simulink model "VMC_3D_Quad_trot"  (R2017a)
settings: Solver=VariableStepAuto  StartTime=0.0  StopTime=20  RelTol=1e-3
model workspace (MATLAB code in the model file):
  | npt=4;  % 接触点个数
  | model = batery_quadruped(npt);
  | f0=zeros(6,1);
  | vx_init=0;
  | x_init = [1;0;0;0; 0;0;1.1; 0;0;0;...
  |           vx_init;0;0]; % initial state
  | q_init = [0;0.5857;-1.1714;0;0.5857;-1.1714;...
  |           0;0.5857;-1.1714;0;0.5857;-1.1714];
  | %q_init = [0;0.7227;-1.4454;0;0.7227;-1.4454;...
  |  %         0;0.7227;-1.4454;0;0.7227;-1.4454];
  | %qd_init= [-2.061;-0.4906];
undefined symbols (not defined in the file or in its folder): batery_quadruped, CalHipVel, CalState, fbanim, FootPUnderHip, Fpt, GaitGenerator, gcontact, gcPosVel, LateralForce, VMC3D
libraries: simulink x4
settings Model: Creator=Jack Lee  LastModifiedBy=jackLee

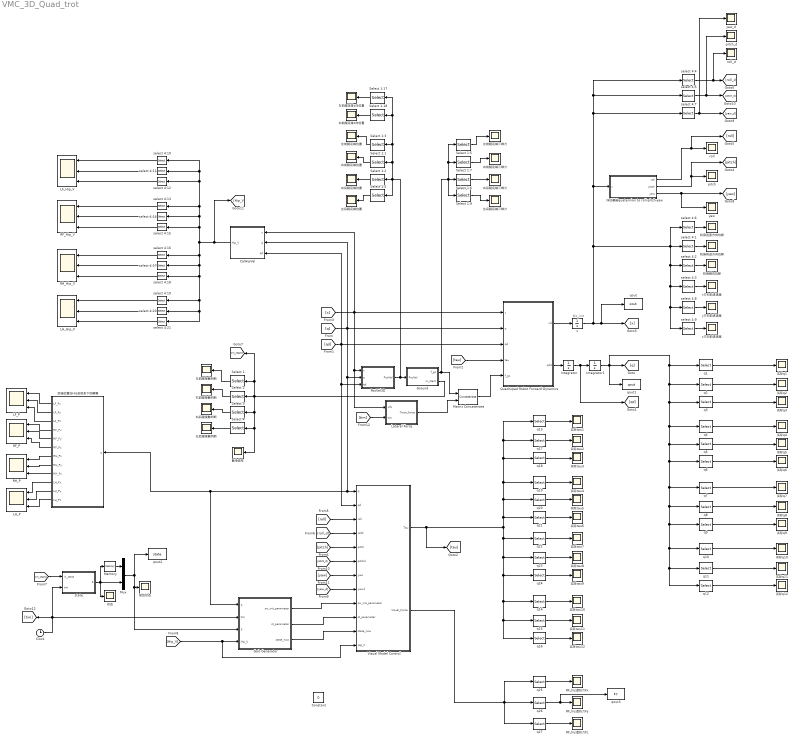
== system VMC_3D_Quad_trot ==
  note: 有x_init
  CalHipVel : Subsystem
  Clock : Clock
  Constant : Constant  Value=0
  Gait Generator : Subsystem
  Ground : Subsystem
  Integrator : Integrator
  Integrator1 : Integrator  InitialCondition=q_init
  LF_Hip_V : Scope  NumInputPorts=3
  LF_P : Scope  NumInputPorts=3
  LH_Hip_V : Scope  NumInputPorts=3
  LH_P : Scope  NumInputPorts=3
  Lateral Force : Subsystem
  Matrix Concatenate : Concatenate  Mode=Multidimensional array  ConcatenateDimension=2
  Memory : Memory  X0=4
  Mux : Mux  Inputs=2
  PosVel3D : Subsystem
  Quadruped Robot Forward Dynamics : Subsystem
  RF_Hip_V : Scope  NumInputPorts=3
  RF_P : Scope  NumInputPorts=3
  RF_hip虚拟力Fx : Scope
  RF_hip虚拟力Fy : Scope
  RF_hip虚拟力Fz : Scope
  RH_Hip_V : Scope  NumInputPorts=3
  RH_P : Scope  NumInputPorts=3
  Select 1 : Selector  InputPortWidth=4  IndexOptions=Index vector (dialog)  Indices=[1]  OutputSizes=1
  Select 1:1 : Selector  NumberOfDimensions=2  InputPortWidth=6  IndexOptions=Index vector (dialog),Index vector (dialog)  Indices=[1 2 3],2  OutputSizes=1,1
  Select 1:17 : Selector  NumberOfDimensions=2  InputPortWidth=6  IndexOptions=Index vector (dialog),Index vector (dialog)  Indices=[3],1  OutputSizes=1,1
  Select 1:18 : Selector  NumberOfDimensions=2  InputPortWidth=6  IndexOptions=Index vector (dialog),Index vector (dialog)  Indices=[3],2  OutputSizes=1,1
  Select 1:2 : Selector  NumberOfDimensions=2  InputPortWidth=6  IndexOptions=Index vector (dialog),Index vector (dialog)  Indices=[1 2 3],3  OutputSizes=1,1
  Select 1:3 : Selector  NumberOfDimensions=2  InputPortWidth=6  IndexOptions=Index vector (dialog),Index vector (dialog)  Indices=[1 2 3],1  OutputSizes=1,1
  Select 1:4 : Selector  NumberOfDimensions=2  InputPortWidth=6  IndexOptions=Index vector (dialog),Index vector (dialog)  Indices=[1 2 3],4  OutputSizes=1,1
  Select 1:5 : Selector  NumberOfDimensions=2  InputPortWidth=6  IndexOptions=Index vector (dialog),Index vector (dialog)  Indices=[4 5 6],1  OutputSizes=1,1
  Select 1:6 : Selector  NumberOfDimensions=2  InputPortWidth=6  IndexOptions=Index vector (dialog),Index vector (dialog)  Indices=[4 5 6],3  OutputSizes=1,1
  Select 1:7 : Selector  NumberOfDimensions=2  InputPortWidth=6  IndexOptions=Index vector (dialog),Index vector (dialog)  Indices=[4 5 6],2  OutputSizes=1,1
  Select 1:9 : Selector  NumberOfDimensions=2  InputPortWidth=6  IndexOptions=Index vector (dialog),Index vector (dialog)  Indices=[4 5 6],4  OutputSizes=1,1
  Select 2 : Selector  InputPortWidth=4  IndexOptions=Index vector (dialog)  Indices=[2]  OutputSizes=1
  Select 3 : Selector  InputPortWidth=4  IndexOptions=Index vector (dialog)  Indices=[3]  OutputSizes=1
  Select 4 : Selector  InputPortWidth=4  IndexOptions=Index vector (dialog)  Indices=[4]  OutputSizes=1
  Visual Model Control : Subsystem
  pitch : Scope
  pitch_d : Scope
  q1 : Selector  InputPortWidth=12  IndexOptions=Index vector (dialog)  Indices=1  OutputSizes=1
  q10 : Selector  InputPortWidth=12  IndexOptions=Index vector (dialog)  Indices=10  OutputSizes=1
  q11 : Selector  InputPortWidth=12  IndexOptions=Index vector (dialog)  Indices=11  OutputSizes=1
  q12 : Selector  InputPortWidth=12  IndexOptions=Index vector (dialog)  Indices=12  OutputSizes=1
  q13 : Selector  InputPortWidth=12  IndexOptions=Index vector (dialog)  Indices=1  OutputSizes=1
  q14 : Selector  InputPortWidth=12  IndexOptions=Index vector (dialog)  Indices=10  OutputSizes=1
  q15 : Selector  InputPortWidth=12  IndexOptions=Index vector (dialog)  Indices=11  OutputSizes=1
  q16 : Selector  InputPortWidth=12  IndexOptions=Index vector (dialog)  Indices=12  OutputSizes=1
  q17 : Selector  InputPortWidth=12  IndexOptions=Index vector (dialog)  Indices=2  OutputSizes=1
  q18 : Selector  InputPortWidth=12  IndexOptions=Index vector (dialog)  Indices=3  OutputSizes=1
  q19 : Selector  InputPortWidth=12  IndexOptions=Index vector (dialog)  Indices=4  OutputSizes=1
  q2 : Selector  InputPortWidth=12  IndexOptions=Index vector (dialog)  Indices=2  OutputSizes=1
  q20 : Selector  InputPortWidth=12  IndexOptions=Index vector (dialog)  Indices=5  OutputSizes=1
  q21 : Selector  InputPortWidth=12  IndexOptions=Index vector (dialog)  Indices=6  OutputSizes=1
  q22 : Selector  InputPortWidth=12  IndexOptions=Index vector (dialog)  Indices=7  OutputSizes=1
  q23 : Selector  InputPortWidth=12  IndexOptions=Index vector (dialog)  Indices=8  OutputSizes=1
  q24 : Selector  InputPortWidth=12  IndexOptions=Index vector (dialog)  Indices=9  OutputSizes=1
  q25 : Selector  InputPortWidth=12  IndexOptions=Index vector (dialog)  Indices=4  OutputSizes=1
  q26 : Selector  InputPortWidth=12  IndexOptions=Index vector (dialog)  Indices=5  OutputSizes=1
  q27 : Selector  InputPortWidth=12  IndexOptions=Index vector (dialog)  Indices=6  OutputSizes=1
  q3 : Selector  InputPortWidth=12  IndexOptions=Index vector (dialog)  Indices=3  OutputSizes=1
  q4 : Selector  InputPortWidth=12  IndexOptions=Index vector (dialog)  Indices=4  OutputSizes=1
  q5 : Selector  InputPortWidth=12  IndexOptions=Index vector (dialog)  Indices=5  OutputSizes=1
  q6 : Selector  InputPortWidth=12  IndexOptions=Index vector (dialog)  Indices=6  OutputSizes=1
  q7 : Selector  InputPortWidth=12  IndexOptions=Index vector (dialog)  Indices=7  OutputSizes=1
  q8 : Selector  InputPortWidth=12  IndexOptions=Index vector (dialog)  Indices=8  OutputSizes=1
  q9 : Selector  InputPortWidth=12  IndexOptions=Index vector (dialog)  Indices=9  OutputSizes=1
  qout : ToWorkspace  VariableName=xout  SampleTime=-1
  qout1 : ToWorkspace  VariableName=qout  SampleTime=-1
  qout2 : ToWorkspace  VariableName=state  SampleTime=-1
  qout3 : ToWorkspace  VariableName=FY  SampleTime=-1
  roll : Scope
  roll_d : Scope
  select 4:1 : Selector  InputPortWidth=13  IndexOptions=Index vector (dialog)  Indices=[5]  OutputSizes=1
  select 4:10 : Selector  InputPortWidth=12  IndexOptions=Index vector (dialog)  Indices=[1]  OutputSizes=1
  select 4:11 : Selector  InputPortWidth=12  IndexOptions=Index vector (dialog)  Indices=[2]  OutputSizes=1
  select 4:12 : Selector  InputPortWidth=12  IndexOptions=Index vector (dialog)  Indices=[3]  OutputSizes=1
  select 4:13 : Selector  InputPortWidth=12  IndexOptions=Index vector (dialog)  Indices=[4]  OutputSizes=1
  select 4:14 : Selector  InputPortWidth=12  IndexOptions=Index vector (dialog)  Indices=[5]  OutputSizes=1
  select 4:15 : Selector  InputPortWidth=12  IndexOptions=Index vector (dialog)  Indices=[6]  OutputSizes=1
  select 4:16 : Selector  InputPortWidth=12  IndexOptions=Index vector (dialog)  Indices=[7]  OutputSizes=1
  select 4:17 : Selector  InputPortWidth=12  IndexOptions=Index vector (dialog)  Indices=[8]  OutputSizes=1
  select 4:18 : Selector  InputPortWidth=12  IndexOptions=Index vector (dialog)  Indices=[9]  OutputSizes=1
  select 4:19 : Selector  InputPortWidth=12  IndexOptions=Index vector (dialog)  Indices=[10]  OutputSizes=1
  select 4:2 : Selector  InputPortWidth=13  IndexOptions=Index vector (dialog)  Indices=[6]  OutputSizes=1
  select 4:20 : Selector  InputPortWidth=12  IndexOptions=Index vector (dialog)  Indices=[11]  OutputSizes=1
  select 4:21 : Selector  InputPortWidth=12  IndexOptions=Index vector (dialog)  Indices=[12]  OutputSizes=1
  select 4:3 : Selector  InputPortWidth=13  IndexOptions=Index vector (dialog)  Indices=[11]  OutputSizes=1
  select 4:4 : Selector  InputPortWidth=13  IndexOptions=Index vector (dialog)  Indices=[8]  OutputSizes=1
  select 4:5 : Selector  InputPortWidth=13  IndexOptions=Index vector (dialog)  Indices=[9]  OutputSizes=1
  select 4:6 : Selector  InputPortWidth=13  IndexOptions=Index vector (dialog)  Indices=[7]  OutputSizes=1
  select 4:7 : Selector  InputPortWidth=13  IndexOptions=Index vector (dialog)  Indices=[10]  OutputSizes=1
  select 4:8 : Selector  InputPortWidth=13  IndexOptions=Index vector (dialog)  Indices=[12]  OutputSizes=1
  select 4:9 : Selector  InputPortWidth=13  IndexOptions=Index vector (dialog)  Indices=[13]  OutputSizes=1
  state : Subsystem
  x : Integrator  InitialCondition=x_init
  x方向前进速度 : Scope
  yaw : Scope
  yaw_d : Scope
  y方向前进速度 : Scope
  z方向前进速度 : Scope
  前后状态 : Scope
  右前腿接触判断 : Scope
  右前腿足端z向位置 : Scope
  右前腿足端三维力 : Scope
  右前腿足端位置 : Scope
  右后腿接触判断 : Scope
  右后腿足端三维力 : Scope
  右后腿足端位置 : Scope
  实际q{1..12} (12 alike) : Scope
  实际tau{1..12} (12 alike) : Scope
  左前腿接触判断 : Scope
  左前腿足端z向位置 : Scope
  左前腿足端三维力 : Scope
  左前腿足端位置 : Scope
  左后腿接触判断 : Scope
  左后腿足端三维力 : Scope
  左后腿足端位置 : Scope
  机身侧向位移 : Scope
  机身前进方向位移 : Scope
  机身竖直方向位移 : Scope
  浮动基座quaternion to roll-pitch-yaw : Subsystem
  状态 : Scope
  触地信号 : Scope
  足端位置在Hip坐标系下的解算 : Subsystem
  wires:
  Quadruped Robot Forward Dynamics/1(xd) -> x/1
  Quadruped Robot Forward Dynamics/2(qdd) -> Integrator/1
  Integrator/1 -> [qd], Integrator1/1
  Ground/1(f_gc) -> Select 1:5/1, Select 1:7/1, Select 1:9/1, Select 1:6/1, Matrix Concatenate/1
  [tau] -> Quadruped Robot Forward Dynamics/4(tau)
  x/1 -> select 4:5/1, select 4:4/1, select 4:7/1, 浮动基座quaternion to roll-pitch-yaw/1(x), select 4:9/1, select 4:8/1, select 4:3/1, select 4:2/1, select 4:6/1, select 4:1/1, qout/1, [x]
  Ground/2(in_ctact) -> [in_ctact], Select 1/1, 触地信号/1, Select 4/1, Select 3/1, Select 2/1
  [x] -> CalHipVel/1(x), Lateral Force/1(xfb), PosVel3D/1(x), Quadruped Robot Forward Dynamics/1(x)
  [qd] -> CalHipVel/3(qd), Visual Model Control/2(qd), PosVel3D/3(qd), Quadruped Robot Forward Dynamics/3(qd)
  PosVel3D/1(PosVel) -> Select 1:18/1, Select 1:17/1, Select 1:3/1, Select 1:1/1, Select 1:4/1, Select 1:2/1, Ground/1(PosVel)
  Select 1:2/1 -> 右后腿足端位置/1
  Select 1:4/1 -> 左后腿足端位置/1
  Select 1:1/1 -> 右前腿足端位置/1
  Select 1:3/1 -> 左前腿足端位置/1
  Select 1:5/1 -> 左前腿足端三维力/1
  Select 1:7/1 -> 右前腿足端三维力/1
  Select 1:6/1 -> 右后腿足端三维力/1
  Select 1:9/1 -> 左后腿足端三维力/1
  Select 1/1 -> 左前腿接触判断/1
  Select 2/1 -> 右前腿接触判断/1
  Select 3/1 -> 右后腿接触判断/1
  Select 4/1 -> 左后腿接触判断/1
  select 4:6/1 -> 机身竖直方向位移/1
  q12/1 -> 实际q12/1
  q11/1 -> 实际q11/1
  q10/1 -> 实际q10/1
  q9/1 -> 实际q9/1
  q8/1 -> 实际q8/1
  q7/1 -> 实际q7/1
  q6/1 -> 实际q6/1
  q5/1 -> 实际q5/1
  q4/1 -> 实际q4/1
  q3/1 -> 实际q3/1
  q2/1 -> 实际q2/1
  Integrator1/1 -> q12/1, q11/1, q10/1, q9/1, q8/1, q7/1, q6/1, q5/1, q4/1, q3/1, q2/1, q1/1, qout1/1, [q]
  q18/1 -> 实际tau3/1
  q24/1 -> 实际tau9/1
  q22/1 -> 实际tau7/1
  q16/1 -> 实际tau12/1
  q17/1 -> 实际tau2/1
  q20/1 -> 实际tau5/1
  q21/1 -> 实际tau6/1
  q23/1 -> 实际tau8/1
  Visual Model Control/1(Tau) -> [tau], q16/1, q15/1, q14/1, q24/1, q23/1, q22/1, q13/1, q17/1, q18/1, q19/1, q20/1, q21/1
  q14/1 -> 实际tau10/1
  q19/1 -> 实际tau4/1
  q13/1 -> 实际tau1/1
  q15/1 -> 实际tau11/1
  select 4:1/1 -> 机身前进方向位移/1
  Select 1:18/1 -> 右前腿足端z向位置/1
  Select 1:17/1 -> 左前腿足端z向位置/1
  select 4:3/1 -> x方向前进速度/1
  浮动基座quaternion to roll-pitch-yaw/2(pitch) -> [pitch], pitch/1
  浮动基座quaternion to roll-pitch-yaw/1(roll) -> [roll], roll/1
  浮动基座quaternion to roll-pitch-yaw/3(yaw) -> [yaw], yaw/1
  select 4:4/1 -> roll_d/1, [roll_d]
  q1/1 -> 实际q1/1
  [in_ctact] -> state/1(in_ctact)
  state/1(S) -> Memory/1, Mux/2, 状态/1
  select 4:5/1 -> pitch_d/1, [pitch_d]
  select 4:7/1 -> yaw_d/1, [yaw_d]
  [roll] -> Visual Model Control/3(roll)
  [roll_d] -> Visual Model Control/4(rolld)
  [pitch] -> Visual Model Control/5(pitch)
  [Hip_V] -> Visual Model Control/12(Hip_V), Gait Generator/4(Hip_V)
  [q] -> CalHipVel/2(q), Gait Generator/1(q), 足端位置在Hip坐标系下的解算/1(q), Visual Model Control/1(q), PosVel3D/2(q), Quadruped Robot Forward Dynamics/2(q)
  Gait Generator/1(sw_init_parameter) -> Visual Model Control/9(sw_init_parameter)
  Gait Generator/2(st_parameter) -> Visual Model Control/10(st_parameter)
  Gait Generator/3(state_now) -> Visual Model Control/11(state_now)
  Clock/1 -> [tim], state/2(tim), Gait Generator/2(tim)
  Mux/1 -> qout2/1, 前后状态/1, Gait Generator/3(S)
  Memory/1 -> Mux/1
  [yaw_d] -> Visual Model Control/8(yawd)
  [pitch_d] -> Visual Model Control/6(pitchd)
  [yaw] -> Visual Model Control/7(yaw)
  select 4:9/1 -> z方向前进速度/1
  足端位置在Hip坐标系下的解算/1(LF_Px) -> LF_P/1
  足端位置在Hip坐标系下的解算/2(LF_Py) -> LF_P/2
  足端位置在Hip坐标系下的解算/3(LF_Pz) -> LF_P/3
  足端位置在Hip坐标系下的解算/4(RF_Px) -> RF_P/1
  足端位置在Hip坐标系下的解算/5(RF_Py) -> RF_P/2
  足端位置在Hip坐标系下的解算/6(RF_Pz) -> RF_P/3
  足端位置在Hip坐标系下的解算/7(RH_Px) -> RH_P/1
  足端位置在Hip坐标系下的解算/8(RH_Py) -> RH_P/2
  足端位置在Hip坐标系下的解算/9(RH_Pz) -> RH_P/3
  足端位置在Hip坐标系下的解算/12(LH_Pz) -> LH_P/3
  足端位置在Hip坐标系下的解算/11(LH_Py) -> LH_P/2
  足端位置在Hip坐标系下的解算/10(LH_Px) -> LH_P/1
  select 4:2/1 -> 机身侧向位移/1
  select 4:8/1 -> y方向前进速度/1
  select 4:10/1 -> LF_Hip_V/1
  select 4:12/1 -> LF_Hip_V/3
  select 4:11/1 -> LF_Hip_V/2
  select 4:15/1 -> RF_Hip_V/3
  select 4:13/1 -> RF_Hip_V/1
  select 4:14/1 -> RF_Hip_V/2
  select 4:18/1 -> RH_Hip_V/3
  select 4:16/1 -> RH_Hip_V/1
  select 4:17/1 -> RH_Hip_V/2
  select 4:21/1 -> LH_Hip_V/3
  select 4:19/1 -> LH_Hip_V/1
  CalHipVel/1(Hip_V) -> [Hip_V], select 4:15/1, select 4:13/1, select 4:12/1, select 4:11/1, select 4:10/1, select 4:14/1, select 4:17/1, select 4:18/1, select 4:19/1, select 4:20/1, select 4:21/1, select 4:16/1
  select 4:20/1 -> LH_Hip_V/2
  [tim] -> Lateral Force/2(tim)
  Lateral Force/1(Torso_force) -> Matrix Concatenate/2
  Matrix Concatenate/1 -> Quadruped Robot Forward Dynamics/5(f_gc)
  Visual Model Control/2(Visual_Force) -> q27/1, q25/1, q26/1
  q27/1 -> RF_hip虚拟力Fz/1
  q26/1 -> qout3/1, RF_hip虚拟力Fy/1
  q25/1 -> RF_hip虚拟力Fx/1

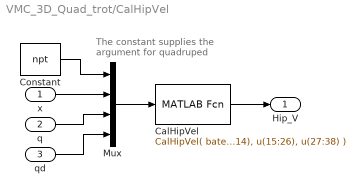
== system VMC_3D_Quad_trot/CalHipVel ==
  note: The constant supplies the
      | argument for quadruped
  x : Inport
  q : Inport  Port=2
  qd : Inport  Port=3
  CalHipVel : MATLABFcn  MATLABFcn=CalHipVel( batery_quadruped(u(1)), u(2:14), u(15:26), u(27:38) )  OutputDimensions=[12 1]  OutputSignalType=real  Output1D=off
  Constant : Constant  Value=npt
  Mux : Mux
  Hip_V : Outport
  wires:
  CalHipVel/1 -> Hip_V/1
  Mux/1 -> CalHipVel/1
  x/1 -> Mux/2
  Constant/1 -> Mux/1
  q/1 -> Mux/3
  qd/1 -> Mux/4

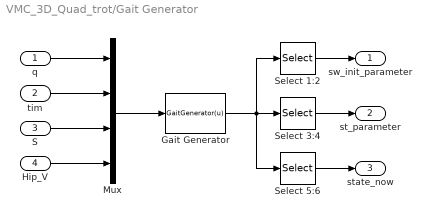
== system VMC_3D_Quad_trot/Gait Generator ==
  q : Inport
  tim : Inport  Port=2
  S : Inport  Port=3
  Hip_V : Inport  Port=4
  Gait Generator : MATLABFcn  MATLABFcn=GaitGenerator(u)  OutputDimensions=[32 1]  OutputSignalType=real  Output1D=off
  Mux : Mux
  Select 1:2 : Selector  InputPortWidth=32  IndexOptions=Index vector (dialog)  Indices=[1:21]  OutputSizes=1
  Select 3:4 : Selector  InputPortWidth=32  IndexOptions=Index vector (dialog)  Indices=[22:31]  OutputSizes=1
  Select 5:6 : Selector  InputPortWidth=32  IndexOptions=Index vector (dialog)  Indices=[32]  OutputSizes=1
  sw_init_parameter : Outport
  st_parameter : Outport  Port=2
  state_now : Outport  Port=3
  wires:
  q/1 -> Mux/1
  Select 1:2/1 -> sw_init_parameter/1
  Select 3:4/1 -> st_parameter/1
  Select 5:6/1 -> state_now/1
  Mux/1 -> Gait Generator/1
  Gait Generator/1 -> Select 5:6/1, Select 1:2/1, Select 3:4/1
  tim/1 -> Mux/2
  S/1 -> Mux/3
  Hip_V/1 -> Mux/4

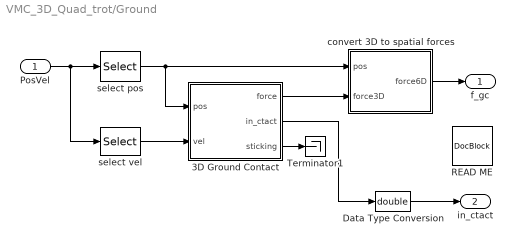
== system VMC_3D_Quad_trot/Ground ==
  PosVel : Inport
  3D Ground Contact : Subsystem  mask(3D Nonlinear Ground Contact with Friction){K=5e5, D=2000, mu=0.7, np=npt}
      mask prompts: K "Stiffness (K)"; D "Damping (D)"; mu "Coefficient of Friction (mu)"; np "Number of Contact Points"
      mask help:
      | Given two 3xnp arrays containing contact-point positions and
      | velocities, calculate the 3xnp array of ground-reaction forces
      | acting on those points. Also calculate 1xnp boolean vectors
      | in_ctact (true if normal force >0) and sticking (true if inside
      | or on boundary of friction cone).  Zero-crossing detection is
      | enabled at both make/break contact and stick/slip transitions.
  Data Type Conversion : DataTypeConversion  OutDataTypeStr=double
  READ ME : simulink/Model-Wide Utilities/DocBlock  DocumentType=Text
      content=|
      | This subsystem implements the Simulink ground-contact model in 3D.  The
      | input is a 6x(npt) matrix such that column i contains the 3D position (top
      | 3 elements) and linear velocity (bottom 3 elements) of ground-contact
      | point number i (i.e., the i^th point defined in the "gc" field of the
      | system model data structure).  The output is a 6x(npt) matrix such that
      | column i is the spatial force acting on point number i.  All quantities
      | are expressed in base (body 0) coordinates.
      |
      | The first thing that happens is that the input matrix is split into
      | separate position and velocity matrices.  Both are then sent to the "3D
      | Ground Contact" subsystem, which calculates the force acting on each
      | point.  The "force" output is a 3x(npt) matrix of linear forces, which is
      | converted to a matrix of spatial forces by the final block in the
      | subsystem.  The other two outputs are 1x(npt) arrays of Boolean variables
      | such that in_ctact(i) is true if point i is in contact with the ground
      | (meaning that it is experiencing a nonzero force) and sticking(i) is true
      | if point i is sticking (due to friction) to the ground.
      |
      | The subsystem "3D Ground Contact" is a masked subsystem.  If you
      | double-click on this block then you will get a dialog window displaying
      | the following parameters: Stiffness (K), Damping (D), coefficient of
      | friction (mu), and Number of Contact Points.  The first three must be
      | strictly-positive scalars, and the fourth must equal the number of points
      | defined in the "gc" field of the system model data structure.  The current
      | settings of K, D and mu correspond to a soft, very slippery plastic
      | surface.  Increasing K will make it harder, and increasing the ratio K/D
      | will make it bouncier, but be aware that both increase the stiffness of
      | the differential equations that Simulink is solving, meaning that Simulink
      | will be forced to take smaller steps.  A typical value of mu for a safe
      | (non-slip) floor is 0.5.
      |
      | To see how this subsystem is implemented, you will have to look under the
      | mask.  You can do that by right-clicking on the block and selecting the
      | menu option "Look Under Mask".  There, you will find that this block is
      | based on the function gcontact, and you will also find a bit more
      | documentation.
  Terminator1 : Terminator
  convert 3D to spatial forces : Subsystem
  select pos : Selector  NumberOfDimensions=2  InputPortWidth=3  IndexOptions=Index vector (dialog),Select all  Indices=[1 2 3],1  OutputSizes=1,1
  select vel : Selector  NumberOfDimensions=2  InputPortWidth=3  IndexOptions=Index vector (dialog),Select all  Indices=[4 5 6],1  OutputSizes=1,1
  f_gc : Outport
  in_ctact : Outport  Port=2
  wires:
  PosVel/1 -> select pos/1, select vel/1
  select pos/1 -> convert 3D to spatial forces/1(pos), 3D Ground Contact/1(pos)
  convert 3D to spatial forces/1(force6D) -> f_gc/1
  select vel/1 -> 3D Ground Contact/2(vel)
  3D Ground Contact/1(force) -> convert 3D to spatial forces/2(force3D)
  3D Ground Contact/3(sticking) -> Terminator1/1
  3D Ground Contact/2(in_ctact) -> Data Type Conversion/1
  Data Type Conversion/1 -> in_ctact/1

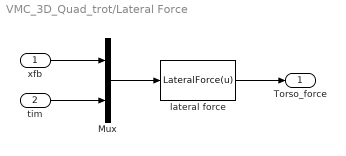
== system VMC_3D_Quad_trot/Lateral Force ==
  xfb : Inport
  tim : Inport  Port=2
  Mux : Mux  Inputs=2
  lateral force : MATLABFcn  MATLABFcn=LateralForce(u)  OutputDimensions=[6 1]  OutputSignalType=real  Output1D=off
  Torso_force : Outport
  wires:
  lateral force/1 -> Torso_force/1
  Mux/1 -> lateral force/1
  xfb/1 -> Mux/1
  tim/1 -> Mux/2

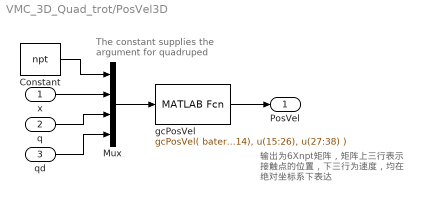
== system VMC_3D_Quad_trot/PosVel3D ==
  note: 输出为6Xnpt矩阵，矩阵上三行表示
      | 接触点的位置，下三行为速度，均在
      | 绝对坐标系下表达
  note: The constant supplies the
      | argument for quadruped
  x : Inport
  q : Inport  Port=2
  qd : Inport  Port=3
  Constant : Constant  Value=npt
  Mux : Mux
  gcPosVel : MATLABFcn  MATLABFcn=gcPosVel( batery_quadruped(u(1)), u(2:14), u(15:26), u(27:38) )  OutputDimensions=[6 npt]  OutputSignalType=real  Output1D=off
  PosVel : Outport
  wires:
  gcPosVel/1 -> PosVel/1
  Mux/1 -> gcPosVel/1
  x/1 -> Mux/2
  Constant/1 -> Mux/1
  q/1 -> Mux/3
  qd/1 -> Mux/4

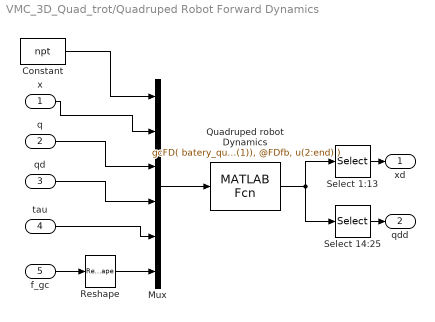
== system VMC_3D_Quad_trot/Quadruped Robot Forward Dynamics ==
  x : Inport
  q : Inport  Port=2
  qd : Inport  Port=3
  tau : Inport  Port=4
  f_gc : Inport  Port=5
  Constant : Constant  Value=npt
  Mux : Mux  Inputs=6
  Quadruped robot Dynamics : MATLABFcn  MATLABFcn=gcFD( batery_quadruped(u(1)), @FDfb, u(2:end) )  OutputDimensions=[25 1]  OutputSignalType=real  Output1D=off
  Reshape : Reshape  OutputDimensionality=Column vector (2-D)
  Select 14:25 : Selector  InputPortWidth=25  IndexOptions=Index vector (dialog)  Indices=[14 15 16 17 18 19 20 21 22 23 24 25]  OutputSizes=1
  Select 1:13 : Selector  InputPortWidth=25  IndexOptions=Index vector (dialog)  Indices=[1 2 3 4 5 6 7 8 9 10 11 12 13]  OutputSizes=1
  xd : Outport
  qdd : Outport  Port=2
  wires:
  f_gc/1 -> Reshape/1
  Mux/1 -> Quadruped robot Dynamics/1
  Reshape/1 -> Mux/6
  x/1 -> Mux/2
  Constant/1 -> Mux/1
  Select 14:25/1 -> qdd/1
  Select 1:13/1 -> xd/1
  Quadruped robot Dynamics/1 -> Select 14:25/1, Select 1:13/1
  q/1 -> Mux/3
  qd/1 -> Mux/4
  tau/1 -> Mux/5

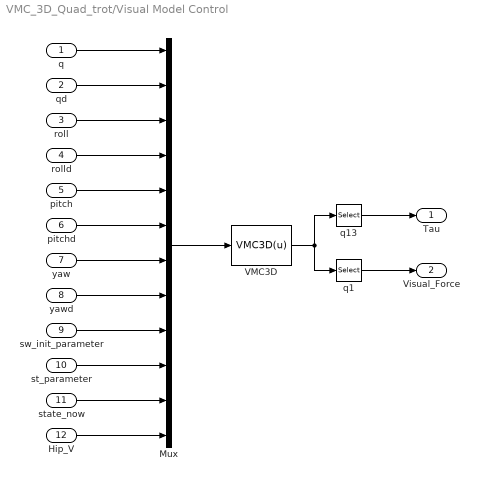
== system VMC_3D_Quad_trot/Visual Model Control ==
  q : Inport
  qd : Inport  Port=2
  roll : Inport  Port=3
  rolld : Inport  Port=4
  pitch : Inport  Port=5
  pitchd : Inport  Port=6
  yaw : Inport  Port=7
  yawd : Inport  Port=8
  sw_init_parameter : Inport  Port=9
  st_parameter : Inport  Port=10
  state_now : Inport  Port=11
  Hip_V : Inport  Port=12
  Mux : Mux  Inputs=12
  VMC3D : MATLABFcn  MATLABFcn=VMC3D(u)  OutputDimensions=[24 1]  OutputSignalType=real  Output1D=off
  q1 : Selector  InputPortWidth=24  IndexOptions=Index vector (dialog)  Indices=[13:24]  OutputSizes=1
  q13 : Selector  InputPortWidth=24  IndexOptions=Index vector (dialog)  Indices=[1:12]  OutputSizes=1
  Tau : Outport
  Visual_Force : Outport  Port=2
  wires:
  q/1 -> Mux/1
  roll/1 -> Mux/3
  pitch/1 -> Mux/5
  Mux/1 -> VMC3D/1
  qd/1 -> Mux/2
  rolld/1 -> Mux/4
  pitchd/1 -> Mux/6
  yaw/1 -> Mux/7
  yawd/1 -> Mux/8
  sw_init_parameter/1 -> Mux/9
  st_parameter/1 -> Mux/10
  state_now/1 -> Mux/11
  Hip_V/1 -> Mux/12
  q13/1 -> Tau/1
  q1/1 -> Visual_Force/1
  VMC3D/1 -> q13/1, q1/1

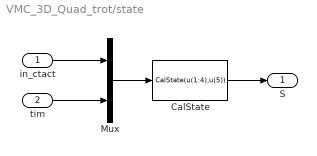
== system VMC_3D_Quad_trot/state ==
  in_ctact : Inport
  tim : Inport  Port=2
  CalState : MATLABFcn  MATLABFcn=CalState(u(1:4),u(5))  OutputDimensions=1  OutputSignalType=real  Output1D=off
  Mux : Mux  Inputs=2
  S : Outport
  wires:
  CalState/1 -> S/1
  Mux/1 -> CalState/1
  in_ctact/1 -> Mux/1
  tim/1 -> Mux/2

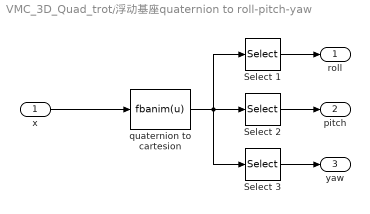
== system VMC_3D_Quad_trot/浮动基座quaternion to roll-pitch-yaw ==
  x : Inport
  Select 1 : Selector  InputPortWidth=6  IndexOptions=Index vector (dialog)  Indices=[4]  OutputSizes=1
  Select 2 : Selector  InputPortWidth=6  IndexOptions=Index vector (dialog)  Indices=[5]  OutputSizes=1
  Select 3 : Selector  InputPortWidth=6  IndexOptions=Index vector (dialog)  Indices=[6]  OutputSizes=1
  "quaternion to cartesion " : MATLABFcn  MATLABFcn=fbanim(u)  OutputDimensions=[6 1]  OutputSignalType=real  Output1D=off
  roll : Outport
  pitch : Outport  Port=2
  yaw : Outport  Port=3
  wires:
  x/1 -> "quaternion to cartesion "/1
  Select 1/1 -> roll/1
  Select 2/1 -> pitch/1
  "quaternion to cartesion "/1 -> Select 1/1, Select 3/1, Select 2/1
  Select 3/1 -> yaw/1

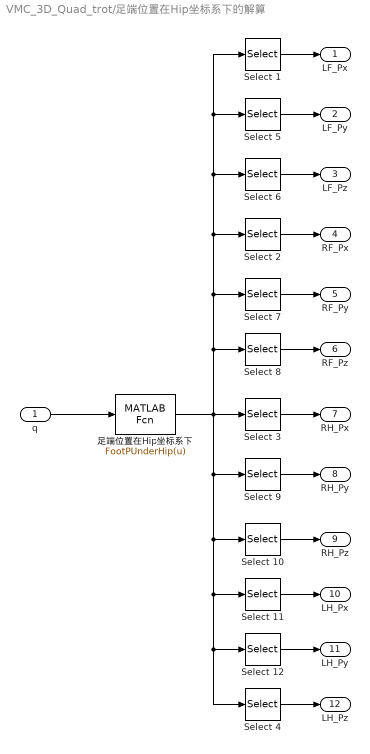
== system VMC_3D_Quad_trot/足端位置在Hip坐标系下的解算 ==
  q : Inport
  Select 1 : Selector  InputPortWidth=12  IndexOptions=Index vector (dialog)  Indices=[1]  OutputSizes=1
  Select 10 : Selector  InputPortWidth=12  IndexOptions=Index vector (dialog)  Indices=[9]  OutputSizes=1
  Select 11 : Selector  InputPortWidth=12  IndexOptions=Index vector (dialog)  Indices=[10]  OutputSizes=1
  Select 12 : Selector  InputPortWidth=12  IndexOptions=Index vector (dialog)  Indices=[11]  OutputSizes=1
  Select 2 : Selector  InputPortWidth=12  IndexOptions=Index vector (dialog)  Indices=[4]  OutputSizes=1
  Select 3 : Selector  InputPortWidth=12  IndexOptions=Index vector (dialog)  Indices=[7]  OutputSizes=1
  Select 4 : Selector  InputPortWidth=12  IndexOptions=Index vector (dialog)  Indices=[12]  OutputSizes=1
  Select 5 : Selector  InputPortWidth=12  IndexOptions=Index vector (dialog)  Indices=[2]  OutputSizes=1
  Select 6 : Selector  InputPortWidth=12  IndexOptions=Index vector (dialog)  Indices=[3]  OutputSizes=1
  Select 7 : Selector  InputPortWidth=12  IndexOptions=Index vector (dialog)  Indices=[5]  OutputSizes=1
  Select 8 : Selector  InputPortWidth=12  IndexOptions=Index vector (dialog)  Indices=[6]  OutputSizes=1
  Select 9 : Selector  InputPortWidth=12  IndexOptions=Index vector (dialog)  Indices=[8]  OutputSizes=1
  足端位置在Hip坐标系下 : MATLABFcn  MATLABFcn=FootPUnderHip(u)  OutputDimensions=[12 1]  OutputSignalType=real  Output1D=off
  LF_Px : Outport
  LF_Py : Outport  Port=2
  LF_Pz : Outport  Port=3
  RF_Px : Outport  Port=4
  RF_Py : Outport  Port=5
  RF_Pz : Outport  Port=6
  RH_Px : Outport  Port=7
  RH_Py : Outport  Port=8
  RH_Pz : Outport  Port=9
  LH_Px : Outport  Port=10
  LH_Py : Outport  Port=11
  LH_Pz : Outport  Port=12
  wires:
  q/1 -> 足端位置在Hip坐标系下/1
  Select 1/1 -> LF_Px/1
  Select 2/1 -> RF_Px/1
  Select 3/1 -> RH_Px/1
  Select 4/1 -> LH_Pz/1
  Select 5/1 -> LF_Py/1
  Select 6/1 -> LF_Pz/1
  Select 7/1 -> RF_Py/1
  Select 8/1 -> RF_Pz/1
  Select 9/1 -> RH_Py/1
  Select 10/1 -> RH_Pz/1
  Select 11/1 -> LH_Px/1
  Select 12/1 -> LH_Py/1
  足端位置在Hip坐标系下/1 -> Select 9/1, Select 10/1, Select 11/1, Select 12/1, Select 4/1, Select 3/1, Select 8/1, Select 7/1, Select 6/1, Select 5/1, Select 1/1, Select 2/1

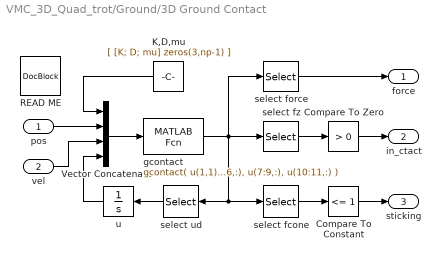
== system VMC_3D_Quad_trot/Ground/3D Ground Contact ==
  pos : Inport
  vel : Inport  Port=2
  Compare To Constant : simulink/Logic and Bit Operations/Compare To Constant  relop=<=  const=1  OutDataTypeStr=boolean
  Compare To Zero : simulink/Logic and Bit Operations/Compare To Zero  relop=>  OutDataTypeStr=boolean
  K,D,mu : Constant  Value=[ [K; D; mu] zeros(3,np-1) ]  VectorParams1D=off
  READ ME : simulink/Model-Wide Utilities/DocBlock  DocumentType=Text
      content=|
      | The constant block supplies the parameters K, D and mu to the function
      | gcontact.  This is necessary because K, D and mu are defined in the
      | workspace of this particular masked subsystem, but the executable
      | expression in the "MATLAB Function" block does not have access to this
      | workspace, so the symbols K, D and mu cannot appear directly in the
      | executable expression.
      |
      | The ">0" block and the "<=1" block both have zero-crossing enabled.  The
      | former detects transitions between contact and non-contact, whereas the
      | latter detects transitions between sticking (due to friction) and
      | slipping.  A point can be sticking only if it is also in contact.  A
      | zero-crossing event occurs whenever any one point makes a transition.
      |
      | The state variable, u, is a 2x(np) matrix containing the horizontal
      | component of the local ground deformation for each point.  This quantity
      | is used to calculate the tangential (i.e., frictional) component of the
      | ground reaction force.
      |
      | When a point loses contact, its associated state variable, u(:,i), decays
      | to zero with a time constant of D/K.  If this ratio is small then the
      | corresponding differential equation is fast, and it is necessary to use
      | small integration time steps.  For example, if K=1e6 and D=2000 then
      | D/K=0.002 and u(:,i) decays in proportion to exp(-500t).  Increasing K
      | makes the surface stiffer, and decreasing D/K makes it bouncier, but the
      | latter also makes the post-contact recovery faster.  The degree of
      | bounciness depends on the mass of the impacting body: a heavier body will
      | bounce more.
      |
      | To adapt this subsystem to work in 2D, the only things that change are the
      | row dimensions of various matrices.  You will have to alter the row
      | selections in the executable expression in the "MATLAB Function" block,
      | and also the dimensions of its output matrix, and you will have to change
      | the row selections in the various "select" blocks.
      |
      | For more information, see "The Simulink Ground Contact Model" in the
      | spatial_v2 documentation directory.
  Vector Concatenate : Concatenate  NumInputs=4  Mode=Multidimensional array
  gcontact : MATLABFcn  MATLABFcn=gcontact( u(1,1), u(2,1), u(3,1), u(4:6,:), u(7:9,:), u(10:11,:) )  OutputDimensions=[6 np]  OutputSignalType=real  Output1D=off
  select fcone : Selector  NumberOfDimensions=2  InputPortWidth=3  IndexOptions=Index vector (dialog),Select all  Indices=[6],1  OutputSizes=1,1
  select force : Selector  NumberOfDimensions=2  InputPortWidth=3  IndexOptions=Index vector (dialog),Select all  Indices=[1 2 3],1  OutputSizes=1,1
  select fz : Selector  NumberOfDimensions=2  InputPortWidth=3  IndexOptions=Index vector (dialog),Select all  Indices=[3],1  OutputSizes=1,1
  select ud : Selector  NumberOfDimensions=2  InputPortWidth=3  IndexOptions=Index vector (dialog),Select all  Indices=[4 5],1  OutputSizes=1,1
  u : Integrator
  force : Outport
  in_ctact : Outport  Port=2
  sticking : Outport  Port=3
  wires:
  Vector Concatenate/1 -> gcontact/1
  select ud/1 -> u/1
  gcontact/1 -> select fz/1, select ud/1, select fcone/1, select force/1
  select force/1 -> force/1
  select fz/1 -> Compare To Zero/1
  Compare To Zero/1 -> in_ctact/1
  select fcone/1 -> Compare To Constant/1
  Compare To Constant/1 -> sticking/1
  u/1 -> Vector Concatenate/4
  vel/1 -> Vector Concatenate/3
  pos/1 -> Vector Concatenate/2
  K,D,mu/1 -> Vector Concatenate/1

== system VMC_3D_Quad_trot/Ground/convert 3D to spatial forces ==
  note: calculate a 6*npt matrix of spatial force vectors (one per column)
      | from a 3*npt matrix of position vectors specifying the points
      | through which the forces act, and a 3*npt matrix of force vectors
  pos : Inport
  force3D : Inport  Port=2
  Fpt : MATLABFcn  MATLABFcn=Fpt( u(4:6,:), u(1:3,:) )  OutputSignalType=real  Output1D=off
  Matrix Concatenate : Concatenate  Mode=Multidimensional array
  force6D : Outport
  wires:
  force3D/1 -> Matrix Concatenate/2
  pos/1 -> Matrix Concatenate/1
  Matrix Concatenate/1 -> Fpt/1
  Fpt/1 -> force6D/1
